simulink model "task_D_mod"  (R2013b)
settings: Solver=ode45  StartTime=0.0  StopTime=10.0  RelTol=1e-3
values from neighbouring files (symbols this model uses):
  a0 = 8*lamda/(c*ro*(b-a)^2)    [task_A_scr.m]    (also in task_B_scr.m = 8*lamda/(3*c*ro*(b-a)^2); task_C_scr.m = 4*lamda*(2-A1-B1)/(c*ro*(b-a)^2))
  A1 = x(1)    [task_C_scr.m]
  A2 = x(1)    [task_C_scr.m]
  A3 = x(1)    [task_C_scr.m]
  a_b = 30000    [task_C_scr.m]
  b1 = 4*lamda*(A2+B2)/(c*ro*(b-a)^2)    [task_C_scr.m]
  B1 = x(2)    [task_C_scr.m]
  b2 = 4*lamda*(A3+B3)/(c*ro*(b-a)^2)    [task_C_scr.m]
  B2 = x(2)    [task_C_scr.m]
  B3 = x(2)    [task_C_scr.m]
  c_b = 415    [task_C_scr.m]
  k_d = 0.01    [task_D_scr.m]
  k_i = 0.1    [task_D_scr.m]
  k_p = 1    [task_D_scr.m]
  Q_b = 0.0425    [task_C_scr.m]
  ro_b = 1000    [task_C_scr.m]
  T_a = 350    [task_A_scr.m]    (also in task_C_scr.m = 600)
  T_b = 400    [task_A_scr.m]    (also in task_B_scr.m = 350; task_C_scr.m = 300)
undefined symbols (not defined in the file or in its folder): T_0
libraries: simulink x1
settings Model: Creator=Yurii  LastModifiedBy=Yurii

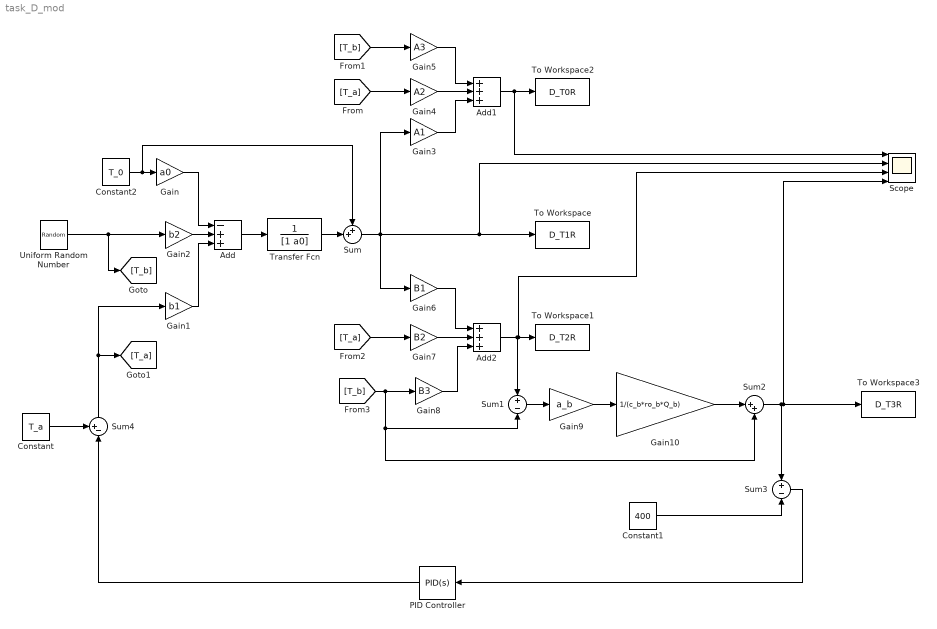
== system task_D_mod ==
  Add : Sum  Inputs=-++
  Add1 : Sum  Inputs=+++
  Add2 : Sum  Inputs=+++
  Constant : Constant  Value=T_a
  Constant1 : Constant  Value=400
  Constant2 : Constant  Value=T_0
  Gain : Gain  Gain=a0
  Gain1 : Gain  Gain=b1
  Gain10 : Gain  Gain=1/(c_b*ro_b*Q_b)
  Gain2 : Gain  Gain=b2
  Gain3 : Gain  Gain=A1
  Gain4 : Gain  Gain=A2
  Gain5 : Gain  Gain=A3
  Gain6 : Gain  Gain=B1
  Gain7 : Gain  Gain=B2
  Gain8 : Gain  Gain=B3
  Gain9 : Gain  Gain=a_b
  PID Controller : simulink/Continuous/PID Controller  Controller=PID  TimeDomain=Continuous-time  SampleTime=1  IntegratorMethod=Forward Euler  FilterMethod=Forward Euler  Form=Parallel  P=k_p  I=k_i  D=k_d  N=100  InitialConditionSource=internal  InitialConditionForIntegrator=0  InitialConditionForFilter=0  ExternalReset=none  LimitOutput=off  UpperSaturationLimit=inf  LowerSaturationLimit=-inf  LinearizeAsGain=on  AntiWindupMode=none  Kb=1  TrackingMode=off  Kt=1  PParamMin=[]  PParamMax=[]  IParamMin=[]  IParamMax=[]  DParamMin=[]  DParamMax=[]  NParamMin=[]  NParamMax=[]  KbParamMin=[]  KbParamMax=[]  KtParamMin=[]  KtParamMax=[]  POutMin=[]  POutMax=[]  IOutMin=[]  IOutMax=[]  DOutMin=[]  DOutMax=[]  NOutMin=[]  NOutMax=[]  KbOutMin=[]  KbOutMax=[]  KtOutMin=[]  KtOutMax=[]  IntegratorOutMin=[]  IntegratorOutMax=[]  FilterOutMin=[]  FilterOutMax=[]  SumOutMin=[]  SumOutMax=[]  SumI1OutMin=[]  SumI1OutMax=[]  SumI2OutMin=[]  SumI2OutMax=[]  SumI3OutMin=[]  SumI3OutMax=[]  SumDOutMin=[]  SumDOutMax=[]  SaturationOutMin=[]  SaturationOutMax=[]  IntegratorContinuousStateAttributes=''  IntegratorStateMustResolveToSignalObject=off  IntegratorRTWStateStorageClass=Auto  FilterContinuousStateAttributes=''  FilterStateMustResolveToSignalObject=off  FilterRTWStateStorageClass=Auto
  Scope : Scope  NumInputPorts=4
      settings: YMin=-5~-5~-5~-5  YMax=5~5~5~5
  Sum : Sum  Inputs=++|
  Sum1 : Sum  Inputs=+|-
  Sum2 : Sum  Inputs=|++
  Sum3 : Sum  Inputs=+|-
  Sum4 : Sum  Inputs=+-|
  To Workspace : ToWorkspace  VariableName=D_T1R  SampleTime=-1  SaveFormat=Timeseries
  To Workspace1 : ToWorkspace  VariableName=D_T2R  SampleTime=-1  SaveFormat=Timeseries
  To Workspace2 : ToWorkspace  VariableName=D_T0R  SampleTime=-1  SaveFormat=Timeseries
  To Workspace3 : ToWorkspace  VariableName=D_T3R  SampleTime=-1  SaveFormat=Timeseries
  Transfer Fcn : TransferFcn  Denominator=[1 a0]
  Uniform Random Number : UniformRandomNumber  Minimum=T_b*0.95  Maximum=T_b*1.05  SampleTime=0
  wires:
  Uniform Random Number/1 -> [T_b], Gain2/1
  Constant2/1 -> Sum/1, Gain/1
  Gain/1 -> Add/1
  Add/1 -> Transfer Fcn/1
  Transfer Fcn/1 -> Sum/2
  Gain1/1 -> Add/3
  Gain2/1 -> Add/2
  Sum/1 -> Gain6/1, Gain3/1, Scope/2, To Workspace/1
  [T_a] -> Gain4/1
  [T_b] -> Gain5/1
  Gain4/1 -> Add1/2
  Gain5/1 -> Add1/1
  Gain3/1 -> Add1/3
  Add1/1 -> Scope/1, To Workspace2/1
  [T_a] -> Gain7/1
  [T_b] -> Sum2/2, Sum1/2, Gain8/1
  Add2/1 -> Scope/3, To Workspace1/1, Sum1/1
  Gain7/1 -> Add2/2
  Gain6/1 -> Add2/1
  Gain8/1 -> Add2/3
  Sum1/1 -> Gain9/1
  Gain9/1 -> Gain10/1
  Gain10/1 -> Sum2/1
  Sum2/1 -> To Workspace3/1, Scope/4, Sum3/1
  Constant1/1 -> Sum3/2
  Sum3/1 -> PID Controller/1
  Constant/1 -> Sum4/1
  PID Controller/1 -> Sum4/2
  Sum4/1 -> [T_a], Gain1/1
